simulink model "lab3s"  (R2022a)
settings: Solver=ode23t  StartTime=0.0  StopTime=Tmdl  FixedStep=Ts  MaxStep=Ts/10  RelTol=1e-3
values from neighbouring files (symbols this model uses):
  J = 3.97381765263    [var_94.mat]
  L = 0.0311    [var_94.mat]
  Psif = 0.125    [var_94.mat]
  R = 17.5665206447    [var_94.mat]
  Ts = 0.0001    [var_94.mat]
  Udc = 48    [var_94.mat]
  Zp = 16    [var_94.mat]
undefined symbols (not defined in the file or in its folder): const, ki, km, kp, T_T, Tq, Trate, u0, um, w
settings Model: Creator=86156  LastModifiedBy=86156
settings ModelReferenceCC: EnableRefExpFcnMdlSchedulingChecks=off
settings RTWCC: Description=Generic Real-Time Target

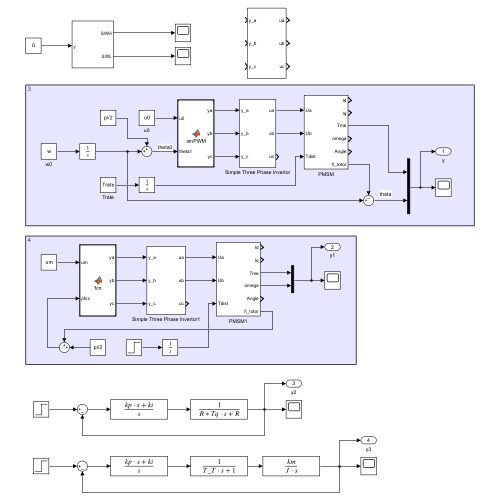
[thumbnail: Simulink's stored preview of the top-level diagram]
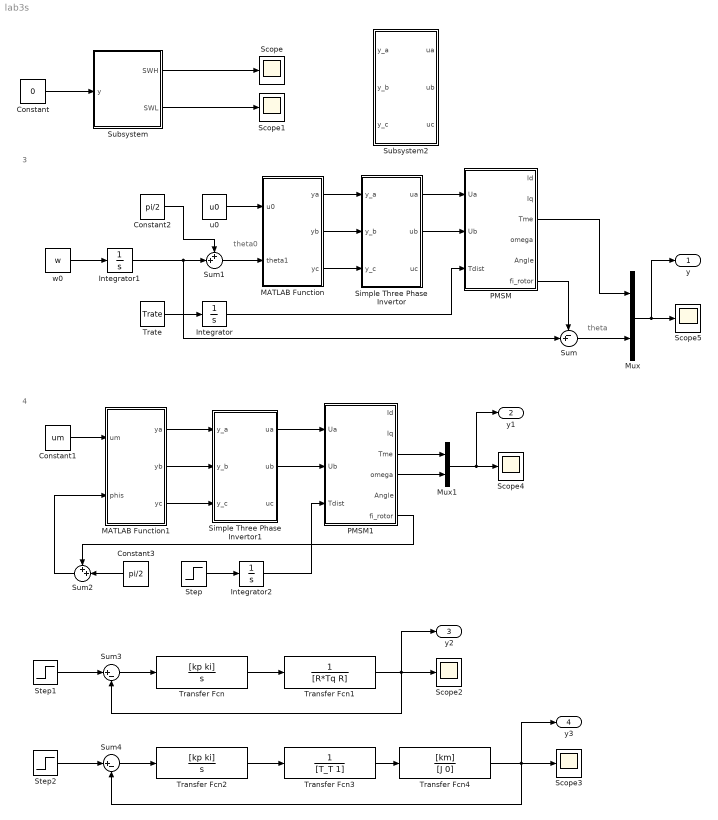
== system lab3s ==
  note: 4
  note: 3
  note: theta
  note: theta0
  Constant : Constant  Value=0
  Constant1 : Constant  Value=um
  Constant2 : Constant  Value=pi/2
  Constant3 : Constant  Value=pi/2
  Integrator : Integrator
  Integrator1 : Integrator  InitialCondition=-1
  Integrator2 : Integrator  InitialCondition=-1
  MATLAB Function : MATLAB Function  TreatAsAtomicUnit=on
  MATLAB Function1 : MATLAB Function  TreatAsAtomicUnit=on
  Mux : Mux  Inputs=2
  Mux1 : Mux  Inputs=2
  PMSM : Subsystem
  PMSM1 : Subsystem
  Scope{,1..5} (6 alike) : Scope
  Simple Three Phase Invertor : Subsystem
  Simple Three Phase Invertor1 : Subsystem
  Step : Step  After=Trate  SampleTime=0
  Step1 : Step  Time=0  SampleTime=0
  Step2 : Step  Time=0  SampleTime=0
  Subsystem : Subsystem
  Subsystem2 : Subsystem
  Sum : Sum  Inputs=-+|
  Sum1 : Sum  Inputs=++|
  Sum2 : Sum  Inputs=++|
  Sum3 : Sum  Inputs=|+-
  Sum4 : Sum  Inputs=|+-
  Transfer Fcn : TransferFcn  Numerator=[kp ki]  Denominator=[1 0]
  Transfer Fcn1 : TransferFcn  Denominator=[R*Tq R]
  Transfer Fcn2 : TransferFcn  Numerator=[kp ki]  Denominator=[1 0]
  Transfer Fcn3 : TransferFcn  Denominator=[T_T 1]
  Transfer Fcn4 : TransferFcn  Numerator=[km]  Denominator=[J 0]
  Trate : Constant  Value=Trate
  u0 : Constant  Value=u0
  w0 : Constant  Value=w
  y : Outport
  y1 : Outport  Port=2
  y2 : Outport  Port=3
  y3 : Outport  Port=4
  wires:
  Subsystem/1(SWH) -> Scope/1
  Subsystem/2(SWL) -> Scope1/1
  Constant/1 -> Subsystem/1(y)
  u0/1 -> MATLAB Function/1(u0)
  Trate/1 -> Integrator/1
  Integrator/1 -> PMSM/3(Tdist)
  PMSM/3(Tme) -> Mux/1
  Mux/1 -> Scope5/1, y/1
  w0/1 -> Integrator1/1
  Sum/1 -> Mux/2
  PMSM/6(fi_rotor) -> Sum/1
  Sum1/1 -> MATLAB Function/2(theta1)
  Integrator1/1 -> Sum/2, Sum1/2
  Simple Three Phase Invertor/1(ua) -> PMSM/1(Ua)
  Simple Three Phase Invertor/2(ub) -> PMSM/2(Ub)
  MATLAB Function/2(yb) -> Simple Three Phase Invertor/2(y_b)
  MATLAB Function/1(ya) -> Simple Three Phase Invertor/1(y_a)
  MATLAB Function/3(yc) -> Simple Three Phase Invertor/3(y_c)
  Constant2/1 -> Sum1/1
  Simple Three Phase Invertor1/1(ua) -> PMSM1/1(Ua)
  Simple Three Phase Invertor1/2(ub) -> PMSM1/2(Ub)
  Constant1/1 -> MATLAB Function1/1(um)
  MATLAB Function1/1(ya) -> Simple Three Phase Invertor1/1(y_a)
  MATLAB Function1/2(yb) -> Simple Three Phase Invertor1/2(y_b)
  MATLAB Function1/3(yc) -> Simple Three Phase Invertor1/3(y_c)
  Constant3/1 -> Sum2/2
  PMSM1/6(fi_rotor) -> Sum2/1
  Sum2/1 -> MATLAB Function1/2(phis)
  Step/1 -> Integrator2/1
  Integrator2/1 -> PMSM1/3(Tdist)
  PMSM1/3(Tme) -> Mux1/1
  Mux1/1 -> Scope4/1, y1/1
  PMSM1/4(omega) -> Mux1/2
  Transfer Fcn/1 -> Transfer Fcn1/1
  Step1/1 -> Sum3/1
  Sum3/1 -> Transfer Fcn/1
  Transfer Fcn1/1 -> y2/1, Sum3/2, Scope2/1
  Transfer Fcn2/1 -> Transfer Fcn3/1
  Step2/1 -> Sum4/1
  Sum4/1 -> Transfer Fcn2/1
  Transfer Fcn3/1 -> Transfer Fcn4/1
  Transfer Fcn4/1 -> y3/1, Sum4/2, Scope3/1

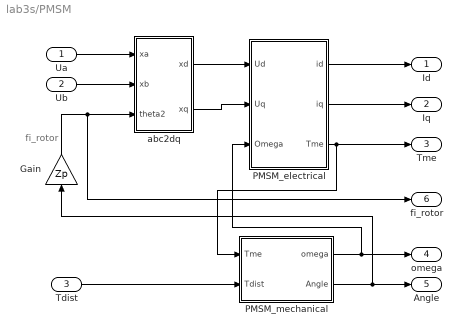
== system lab3s/PMSM ==
  note: fi_rotor
  Ua : Inport
  Ub : Inport  Port=2
  Tdist : Inport  Port=3
  Gain : Gain  Gain=Zp
  "PMSM_electrical " : Subsystem
  PMSM_mechanical : Subsystem
  abc2dq : MATLAB Function  TreatAsAtomicUnit=on
  Id : Outport
  Iq : Outport  Port=2
  Tme : Outport  Port=3
  omega : Outport  Port=4
  Angle : Outport  Port=5
  fi_rotor : Outport  Port=6
  wires:
  "PMSM_electrical "/3(Tme) -> Tme/1, PMSM_mechanical/1(Tme)
  PMSM_mechanical/1(omega) -> "PMSM_electrical "/3(Omega), omega/1
  Tdist/1 -> PMSM_mechanical/2(Tdist)
  abc2dq/1(xd) -> "PMSM_electrical "/1(Ud)
  "PMSM_electrical "/1(id) -> Id/1
  abc2dq/2(xq) -> "PMSM_electrical "/2(Uq)
  Gain/1 -> fi_rotor/1, abc2dq/3(theta2)
  PMSM_mechanical/2(Angle) -> Gain/1, Angle/1
  "PMSM_electrical "/2(iq) -> Iq/1
  Ub/1 -> abc2dq/2(xb)
  Ua/1 -> abc2dq/1(xa)

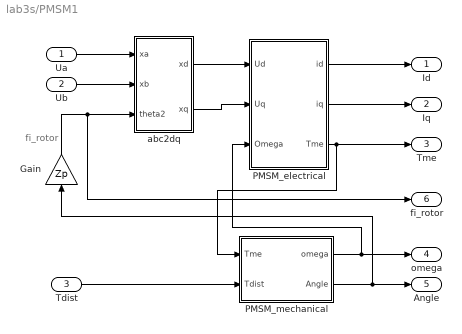
== system lab3s/PMSM1 ==
  note: fi_rotor
  Ua : Inport
  Ub : Inport  Port=2
  Tdist : Inport  Port=3
  Gain : Gain  Gain=Zp
  "PMSM_electrical " : Subsystem
  PMSM_mechanical : Subsystem
  abc2dq : MATLAB Function  TreatAsAtomicUnit=on
  Id : Outport
  Iq : Outport  Port=2
  Tme : Outport  Port=3
  omega : Outport  Port=4
  Angle : Outport  Port=5
  fi_rotor : Outport  Port=6
  wires:
  "PMSM_electrical "/3(Tme) -> Tme/1, PMSM_mechanical/1(Tme)
  PMSM_mechanical/1(omega) -> "PMSM_electrical "/3(Omega), omega/1
  Tdist/1 -> PMSM_mechanical/2(Tdist)
  abc2dq/1(xd) -> "PMSM_electrical "/1(Ud)
  "PMSM_electrical "/1(id) -> Id/1
  abc2dq/2(xq) -> "PMSM_electrical "/2(Uq)
  Gain/1 -> fi_rotor/1, abc2dq/3(theta2)
  PMSM_mechanical/2(Angle) -> Gain/1, Angle/1
  "PMSM_electrical "/2(iq) -> Iq/1
  Ub/1 -> abc2dq/2(xb)
  Ua/1 -> abc2dq/1(xa)

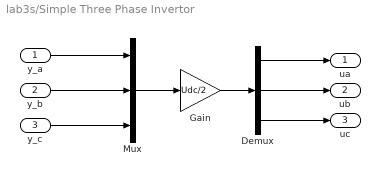
== system lab3s/Simple Three Phase Invertor ==
  y_a : Inport
  y_b : Inport  Port=2
  y_c : Inport  Port=3
  Demux : Demux  Outputs=3
  Gain : Gain  Gain=Udc/2
  Mux : Mux  Inputs=3
  ua : Outport
  ub : Outport  Port=2
  uc : Outport  Port=3
  wires:
  y_a/1 -> Mux/1
  y_b/1 -> Mux/2
  y_c/1 -> Mux/3
  Mux/1 -> Gain/1
  Gain/1 -> Demux/1
  Demux/1 -> ua/1
  Demux/2 -> ub/1
  Demux/3 -> uc/1

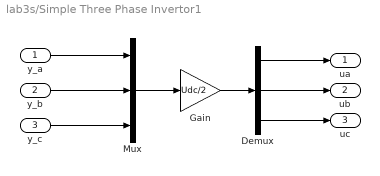
== system lab3s/Simple Three Phase Invertor1 ==
  y_a : Inport
  y_b : Inport  Port=2
  y_c : Inport  Port=3
  Demux : Demux  Outputs=3
  Gain : Gain  Gain=Udc/2
  Mux : Mux  Inputs=3
  ua : Outport
  ub : Outport  Port=2
  uc : Outport  Port=3
  wires:
  y_a/1 -> Mux/1
  y_b/1 -> Mux/2
  y_c/1 -> Mux/3
  Mux/1 -> Gain/1
  Gain/1 -> Demux/1
  Demux/1 -> ua/1
  Demux/2 -> ub/1
  Demux/3 -> uc/1

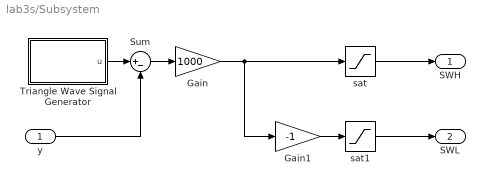
== system lab3s/Subsystem ==
  y : Inport
  Gain : Gain  Gain=1000
  Gain1 : Gain  Gain=-1
  Sum : Sum  Inputs=|+-
  Triangle Wave Signal Generator : Subsystem
  sat : Saturate  UpperLimit=1  LowerLimit=0
  sat1 : Saturate  UpperLimit=1  LowerLimit=0
  SWH : Outport
  SWL : Outport  Port=2
  wires:
  sat/1 -> SWH/1
  Gain/1 -> Gain1/1, sat/1
  Triangle Wave Signal Generator/1(u) -> Sum/1
  Sum/1 -> Gain/1
  sat1/1 -> SWL/1
  y/1 -> Sum/2
  Gain1/1 -> sat1/1

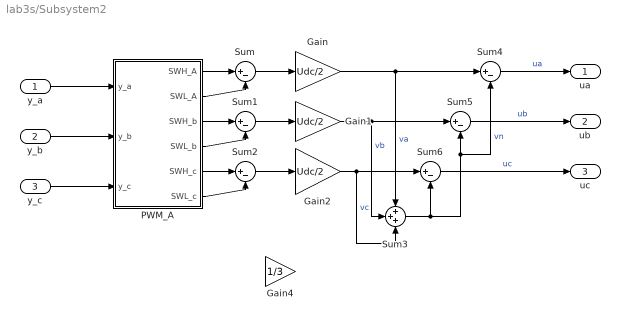
== system lab3s/Subsystem2 ==
  y_a : Inport
  y_b : Inport  Port=2
  y_c : Inport  Port=3
  Gain : Gain  Gain=Udc/2
  Gain1 : Gain  Gain=Udc/2
  Gain2 : Gain  Gain=Udc/2
  Gain4 : Gain  Gain=1/3
  PWM_A : Subsystem
  Sum{,1..2,4..6} (6 alike) : Sum  Inputs=|+-
  Sum3 : Sum  Inputs=+++
  ua : Outport
  ub : Outport  Port=2
  uc : Outport  Port=3
  wires:
  Gain2/1 -> Sum6/1, Sum3/3  "vc"
  PWM_A/4(SWL_b) -> Sum1/2
  y_c/1 -> PWM_A/3(y_c)
  Sum3/1 -> Sum6/2, Sum5/2, Sum4/2  "vn"
  Sum1/1 -> Gain1/1
  PWM_A/5(SWH_c) -> Sum2/1
  Gain1/1 -> Sum3/2, Sum5/1  "vb"
  Gain/1 -> Sum3/1, Sum4/1  "va"
  PWM_A/6(SWL_c) -> Sum2/2
  y_a/1 -> PWM_A/1(y_a)
  PWM_A/3(SWH_b) -> Sum1/1
  Sum2/1 -> Gain2/1
  Sum/1 -> Gain/1
  PWM_A/1(SWH_A) -> Sum/1
  PWM_A/2(SWL_A) -> Sum/2
  Sum6/1 -> uc/1  "uc"
  Sum4/1 -> ua/1  "ua"
  Sum5/1 -> ub/1  "ub"
  y_b/1 -> PWM_A/2(y_b)

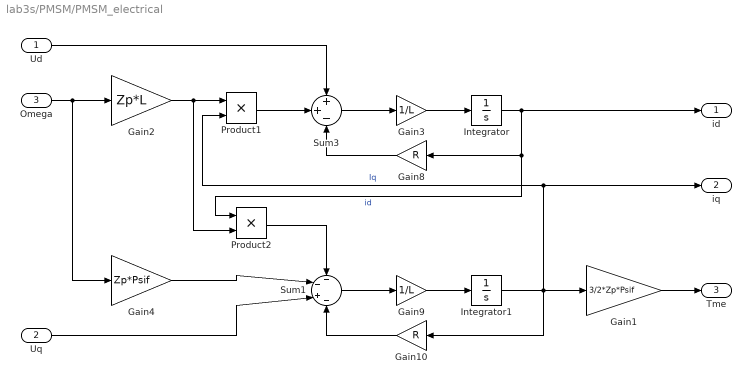
== system lab3s/PMSM/PMSM_electrical  ==
  Ud : Inport
  Uq : Inport  Port=2
  Omega : Inport  Port=3
  Gain1 : Gain  Gain=3/2*Zp*Psif
  Gain10 : Gain  Gain=R
  Gain2 : Gain  Gain=Zp*L
  Gain3 : Gain  Gain=1/L
  Gain4 : Gain  Gain=Zp*Psif
  Gain8 : Gain  Gain=R
  Gain9 : Gain  Gain=1/L
  Integrator : Integrator
  Integrator1 : Integrator
  Product1 : Product
  Product2 : Product
  Sum1 : Sum  Inputs=--+-
  Sum3 : Sum  Inputs=++-
  id : Outport
  iq : Outport  Port=2
  Tme : Outport  Port=3
  wires:
  Integrator/1 -> id/1, Product2/1, Gain8/1  "id"
  Gain2/1 -> Product2/2, Product1/1
  Gain3/1 -> Integrator/1
  Gain10/1 -> Sum1/4
  Gain9/1 -> Integrator1/1
  Gain8/1 -> Sum3/3
  Integrator1/1 -> Gain1/1, Product1/2, iq/1, Gain10/1  "Iq"
  Product2/1 -> Sum1/1
  Sum1/1 -> Gain9/1
  Sum3/1 -> Gain3/1
  Omega/1 -> Gain2/1, Gain4/1
  Product1/1 -> Sum3/2
  Gain1/1 -> Tme/1
  Uq/1 -> Sum1/3
  Gain4/1 -> Sum1/2
  Ud/1 -> Sum3/1

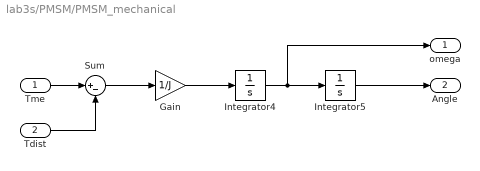
== system lab3s/PMSM/PMSM_mechanical ==
  Tme : Inport
  Tdist : Inport  Port=2
  Gain : Gain  Gain=1/J
  Integrator4 : Integrator
  Integrator5 : Integrator
  Sum : Sum  Inputs=|+-
  omega : Outport
  Angle : Outport  Port=2
  wires:
  Tdist/1 -> Sum/2
  Integrator4/1 -> omega/1, Integrator5/1
  Tme/1 -> Sum/1
  Sum/1 -> Gain/1
  Integrator5/1 -> Angle/1
  Gain/1 -> Integrator4/1

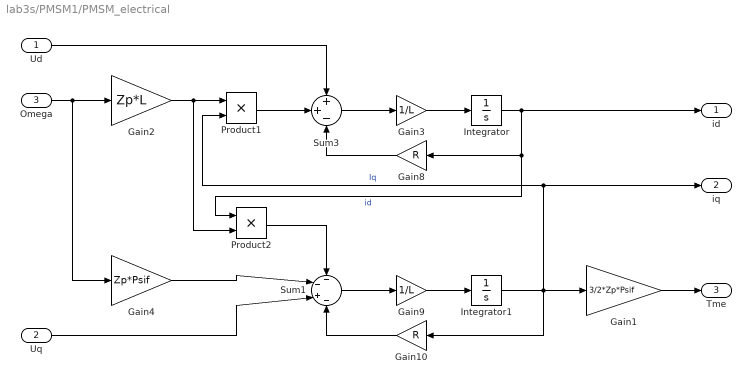
== system lab3s/PMSM1/PMSM_electrical  ==
  Ud : Inport
  Uq : Inport  Port=2
  Omega : Inport  Port=3
  Gain1 : Gain  Gain=3/2*Zp*Psif
  Gain10 : Gain  Gain=R
  Gain2 : Gain  Gain=Zp*L
  Gain3 : Gain  Gain=1/L
  Gain4 : Gain  Gain=Zp*Psif
  Gain8 : Gain  Gain=R
  Gain9 : Gain  Gain=1/L
  Integrator : Integrator
  Integrator1 : Integrator
  Product1 : Product
  Product2 : Product
  Sum1 : Sum  Inputs=--+-
  Sum3 : Sum  Inputs=++-
  id : Outport
  iq : Outport  Port=2
  Tme : Outport  Port=3
  wires:
  Integrator/1 -> id/1, Product2/1, Gain8/1  "id"
  Gain2/1 -> Product2/2, Product1/1
  Gain3/1 -> Integrator/1
  Gain10/1 -> Sum1/4
  Gain9/1 -> Integrator1/1
  Gain8/1 -> Sum3/3
  Integrator1/1 -> Gain1/1, Product1/2, iq/1, Gain10/1  "Iq"
  Product2/1 -> Sum1/1
  Sum1/1 -> Gain9/1
  Sum3/1 -> Gain3/1
  Omega/1 -> Gain2/1, Gain4/1
  Product1/1 -> Sum3/2
  Gain1/1 -> Tme/1
  Uq/1 -> Sum1/3
  Gain4/1 -> Sum1/2
  Ud/1 -> Sum3/1

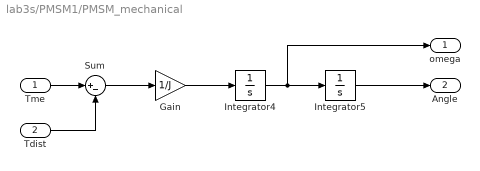
== system lab3s/PMSM1/PMSM_mechanical ==
  Tme : Inport
  Tdist : Inport  Port=2
  Gain : Gain  Gain=1/J
  Integrator4 : Integrator
  Integrator5 : Integrator
  Sum : Sum  Inputs=|+-
  omega : Outport
  Angle : Outport  Port=2
  wires:
  Tdist/1 -> Sum/2
  Integrator4/1 -> omega/1, Integrator5/1
  Tme/1 -> Sum/1
  Sum/1 -> Gain/1
  Integrator5/1 -> Angle/1
  Gain/1 -> Integrator4/1

== system lab3s/Subsystem/Triangle Wave Signal Generator ==
  Constant : Constant  Value=const
  Gain : Gain  Gain=4/Ts
  Integrator : Integrator  InitialCondition=-1
  Pulse Generator : DiscretePulseGenerator  PulseType=Time based  Amplitude=2  Period=Ts  PulseWidth=50
  Sum : Sum  Inputs=|+-
  u : Outport
  wires:
  Sum/1 -> Gain/1
  Gain/1 -> Integrator/1
  Constant/1 -> Sum/2
  Pulse Generator/1 -> Sum/1
  Integrator/1 -> u/1

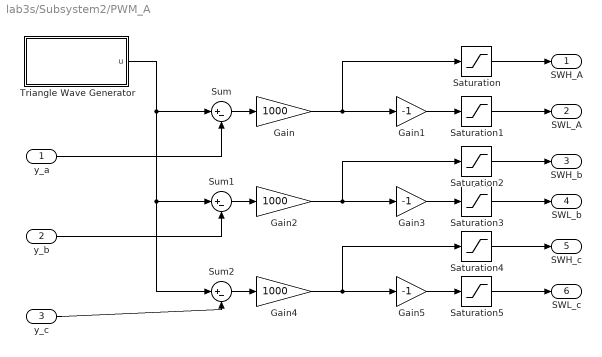
== system lab3s/Subsystem2/PWM_A ==
  y_a : Inport
  y_b : Inport  Port=2
  y_c : Inport  Port=3
  Gain : Gain  Gain=1000
  Gain1 : Gain  Gain=-1
  Gain2 : Gain  Gain=1000
  Gain3 : Gain  Gain=-1
  Gain4 : Gain  Gain=1000
  Gain5 : Gain  Gain=-1
  Saturation{,1..5} (6 alike) : Saturate  UpperLimit=1  LowerLimit=0
  Sum : Sum  Inputs=|+-
  Sum1 : Sum  Inputs=|+-
  Sum2 : Sum  Inputs=|+-
  Triangle Wave Generator : Subsystem
  SWH_A : Outport
  SWL_A : Outport  Port=2
  SWH_b : Outport  Port=3
  SWL_b : Outport  Port=4
  SWH_c : Outport  Port=5
  SWL_c : Outport  Port=6
  wires:
  Gain/1 -> Saturation/1, Gain1/1
  Saturation/1 -> SWH_A/1
  Sum/1 -> Gain/1
  Saturation1/1 -> SWL_A/1
  y_a/1 -> Sum/2
  Gain1/1 -> Saturation1/1
  Gain3/1 -> Saturation3/1
  Gain2/1 -> Saturation2/1, Gain3/1
  Sum1/1 -> Gain2/1
  Saturation3/1 -> SWL_b/1
  y_b/1 -> Sum1/2
  Saturation2/1 -> SWH_b/1
  Sum2/1 -> Gain4/1
  Gain4/1 -> Gain5/1, Saturation4/1
  Gain5/1 -> Saturation5/1
  Triangle Wave Generator/1(u) -> Sum2/1, Sum1/1, Sum/1
  Saturation5/1 -> SWL_c/1
  y_c/1 -> Sum2/2
  Saturation4/1 -> SWH_c/1

== system lab3s/Subsystem2/PWM_A/Triangle Wave Generator ==
  Constant : Constant
  Gain : Gain  Gain=4/Ts
  Integrator : Integrator  InitialCondition=-1
  Pulse Generator : DiscretePulseGenerator  PulseType=Time based  Amplitude=2  Period=Ts  PulseWidth=50
  Sum : Sum  Inputs=|+-
  u : Outport
  wires:
  Integrator/1 -> u/1
  Constant/1 -> Sum/2
  Gain/1 -> Integrator/1
  Pulse Generator/1 -> Sum/1
  Sum/1 -> Gain/1

== matlab function lab3s/MATLAB Function ==
  data: u0 input; ya output; theta1 input; yb output; yc output
function [ya,yb,yc]=sinPWM(u0,theta1)
    ya=u0*sin(theta1);
    yb=u0*sin(theta1-2*pi/3);
    yc=u0*sin(theta1+2*pi/3);

== matlab function lab3s/PMSM/abc2dq ==
  data: xd output; xq output; xa input; xb input; theta2 input
function [xd,xq]=fcn(xa,xb,theta2)

    xd = 2/sqrt(3)*(xa*sin(theta2+pi/3)+xb*sin(theta2));
    xq = 2/sqrt(3)*(xa*cos(theta2+pi/3)+xb*cos(theta2));

== matlab function lab3s/MATLAB Function1 ==
  data: um input; ya output; phis input; yb output; yc output
function [ya,yb,yc]=fcn(um,phis)
    ya=um*sin(phis);
    yb=um*sin(phis-2*pi/3);
    yc=um*sin(phis+2*pi/3);

== matlab function lab3s/PMSM1/abc2dq ==
  data: xd output; xq output; xa input; xb input; theta2 input
function [xd,xq]=fcn(xa,xb,theta2)

    xd = 2/sqrt(3)*(xa*sin(theta2+pi/3)+xb*sin(theta2));
    xq = 2/sqrt(3)*(xa*cos(theta2+pi/3)+xb*cos(theta2));
